simulink model "gcu"  (R2025b)
settings: Solver=FixedStepAuto  StartTime=0.0  StopTime=10.0  RelTol=1e-3
undefined symbols (not defined in the file): controller, luen, quadcop, traj, Ts_gcs, xi0
settings Model: DataDictionary=project.sldd  Creator=Nick  LastModifiedBy=Rakete

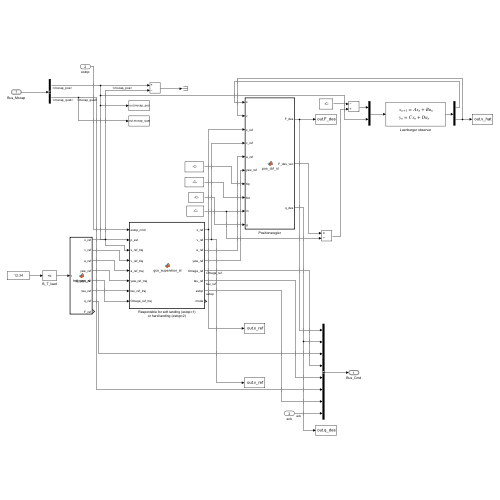
[thumbnail: Simulink's stored preview of the top-level diagram]
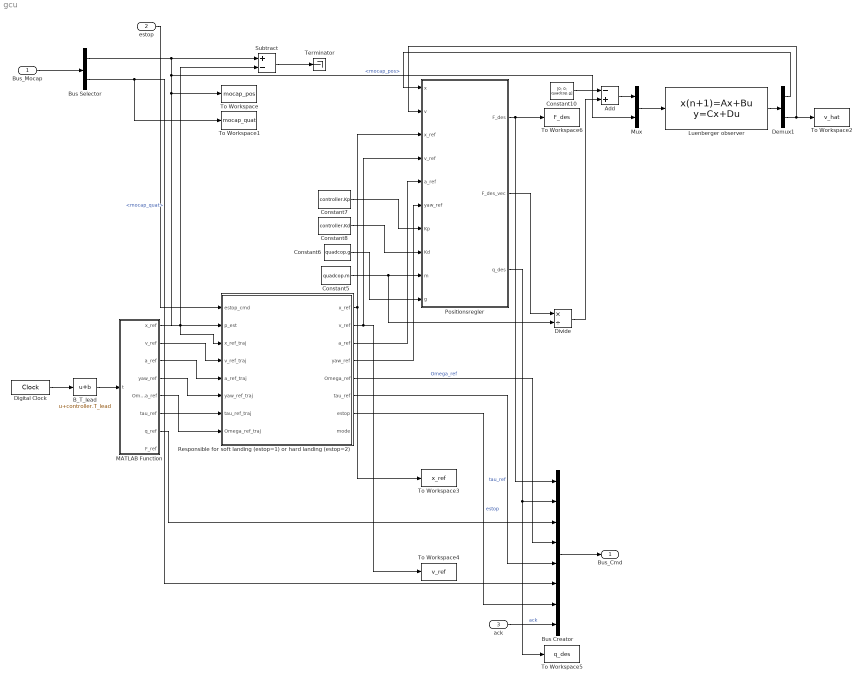
== system gcu ==
  Bus_Mocap : Inport  OutDataTypeStr=Bus: Bus_Mocap
  estop : Inport  Port=2  OutDataTypeStr=uint8
  ack : Inport  Port=3  OutDataTypeStr=boolean  PortDimensions=1
  Add : Sum  Inputs=-+
  B_T_lead : Bias  Bias=controller.T_lead  SaturateOnIntegerOverflow=off
  Bus Creator : BusCreator  Inputs=8  OutDataTypeStr=Bus: Bus_Cmd
      settings: InheritFromInputs=off
  Bus Selector : BusSelector  OutputSignals=mocap_pos,mocap_quat
  Constant10 : Constant  Value=[0; 0; quadcop.g]
  Constant5 : Constant  Value=quadcop.m
  Constant6 : Constant  Value=quadcop.g
  Constant7 : Constant  Value=controller.Kp
  Constant8 : Constant  Value=controller.Kd
  Demux1 : Demux  Outputs=2
  Digital Clock : DigitalClock  SampleTime=Ts_gcs
  Divide : Product  Inputs=*/
  Luenberger observer : DiscreteStateSpace  A=luen.Ad  B=luen.Bd  C=luen.Cd  D=luen.Dd  InitialCondition=xi0  SampleTime=Ts_gcs
  MATLAB Function : MATLAB Function  TreatAsAtomicUnit=on
  Mux : Mux  Inputs=2
  Positionsregler : MATLAB Function  TreatAsAtomicUnit=on
  Responsible for soft landing (estop=1) or hard landing (estop=2) : MATLAB Function  TreatAsAtomicUnit=on  SystemSampleTime=Ts_gcs
  Subtract : Sum  Inputs=+-
  Terminator : Terminator
  To Workspace : ToWorkspace  VariableName=mocap_pos  SaveFormat=Timeseries  SampleTime=Ts_gcs
  To Workspace1 : ToWorkspace  VariableName=mocap_quat  SaveFormat=Timeseries  SampleTime=Ts_gcs
  To Workspace2 : ToWorkspace  VariableName=v_hat  SaveFormat=Timeseries  SampleTime=Ts_gcs
  To Workspace3 : ToWorkspace  VariableName=x_ref  SaveFormat=Timeseries  SampleTime=Ts_gcs
  To Workspace4 : ToWorkspace  VariableName=v_ref  SaveFormat=Timeseries  SampleTime=Ts_gcs
  To Workspace5 : ToWorkspace  VariableName=q_des  SaveFormat=Timeseries  SampleTime=Ts_gcs
  To Workspace6 : ToWorkspace  VariableName=F_des  SaveFormat=Timeseries  SampleTime=Ts_gcs
  Bus_Cmd : Outport  OutDataTypeStr=Bus: Bus_Cmd
  wires:
  Responsible for soft landing (estop=1) or hard landing (estop=2)/7(estop) -> Bus Creator/7  "estop"
  MATLAB Function/2(v_ref) -> Responsible for soft landing (estop=1) or hard landing (estop=2)/4(v_ref_traj)
  Responsible for soft landing (estop=1) or hard landing (estop=2)/3(a_ref) -> Positionsregler/5(a_ref)
  MATLAB Function/6(tau_ref) -> Responsible for soft landing (estop=1) or hard landing (estop=2)/7(tau_ref_traj)
  Digital Clock/1 -> B_T_lead/1
  Bus_Mocap/1 -> Bus Selector/1
  MATLAB Function/1(x_ref) -> Subtract/2, Responsible for soft landing (estop=1) or hard landing (estop=2)/3(x_ref_traj)
  B_T_lead/1 -> MATLAB Function/1(t)
  Add/1 -> Mux/1
  Bus Selector/1 -> Responsible for soft landing (estop=1) or hard landing (estop=2)/2(p_est), To Workspace/1, Mux/2, Subtract/1  "<mocap_pos>"
  Responsible for soft landing (estop=1) or hard landing (estop=2)/6(tau_ref) -> Bus Creator/5  "tau_ref"
  estop/1 -> Responsible for soft landing (estop=1) or hard landing (estop=2)/1(estop_cmd)
  Constant7/1 -> Positionsregler/7(Kp)
  Bus Selector/2 -> Bus Creator/6, To Workspace1/1  "<mocap_quat>"
  MATLAB Function/3(a_ref) -> Responsible for soft landing (estop=1) or hard landing (estop=2)/5(a_ref_traj)
  MATLAB Function/4(yaw_ref) -> Responsible for soft landing (estop=1) or hard landing (estop=2)/6(yaw_ref_traj)
  Responsible for soft landing (estop=1) or hard landing (estop=2)/4(yaw_ref) -> Positionsregler/6(yaw_ref)
  MATLAB Function/5(Omega_ref) -> Responsible for soft landing (estop=1) or hard landing (estop=2)/8(Omega_ref_traj)
  MATLAB Function/7(q_ref) -> Bus Creator/3
  Subtract/1 -> Terminator/1
  Constant8/1 -> Positionsregler/8(Kd)
  Constant6/1 -> Positionsregler/10(g)
  Constant5/1 -> Divide/2, Positionsregler/9(m)
  Responsible for soft landing (estop=1) or hard landing (estop=2)/1(x_ref) -> Positionsregler/3(x_ref), To Workspace3/1
  Responsible for soft landing (estop=1) or hard landing (estop=2)/2(v_ref) -> To Workspace4/1, Positionsregler/4(v_ref)
  Responsible for soft landing (estop=1) or hard landing (estop=2)/5(Omega_ref) -> Bus Creator/4  "Omega_ref"
  Positionsregler/1(F_des) -> Bus Creator/1, To Workspace6/1
  Divide/1 -> Add/2
  Positionsregler/2(F_des_vec) -> Divide/1
  Positionsregler/3(q_des) -> To Workspace5/1, Bus Creator/2
  ack/1 -> Bus Creator/8  "ack"
  Constant10/1 -> Add/1
  Bus Creator/1 -> Bus_Cmd/1
  Mux/1 -> Luenberger observer/1
  Luenberger observer/1 -> Demux1/1
  Demux1/1 -> Positionsregler/1(x)
  Demux1/2 -> Positionsregler/2(v), To Workspace2/1

== matlab function gcu/Positionsregler ==
  data: F_des output; x input; F_des_vec output; v input; x_ref input; v_ref input; a_ref input; yaw_ref input; Kp input; Kd input; m input; g input; q_des output
function [F_des, F_des_vec, q_des] = pos_ctrl_sl(x, v, x_ref, v_ref, a_ref, yaw_ref, Kp, Kd, m, g)
%#codegen
% WRAPPER — code liegt in
% scripts\functions\pos_ctrl.m - dieser Block ruft sie nur auf
[F_des, F_des_vec, q_des] = pos_ctrl(x, v, x_ref, v_ref, a_ref, yaw_ref, Kp, Kd, m, g);
end

== matlab function gcu/MATLAB Function ==
  data: t input; x_ref output; v_ref output; a_ref output; yaw_ref output; Omega_ref output; tau_ref output; q_ref output; F_ref output; traj parameter; quadcop parameter
function [x_ref, v_ref, a_ref, yaw_ref, Omega_ref, tau_ref, q_ref, F_ref] = traj_gen_sl(t, traj, quadcop)
%#codegen
% WRAPPER — code liegt in
% scripts\functions\traj_gen.m - dieser Block ruft sie nur auf
[x_ref, v_ref, a_ref, yaw_ref, Omega_ref, tau_ref, q_ref, F_ref] = traj_gen(t, traj, quadcop);
end

== matlab function gcu/Responsible for soft landing (estop=1) or hard landing (estop=2) ==
  data: estop_cmd input; x_ref output; p_est input; x_ref_traj input; v_ref_traj input; a_ref_traj input; yaw_ref_traj input; v_ref output; a_ref output; yaw_ref output; Omega_ref output; tau_ref output; estop output; mode output; tau_ref_traj input; supervisor parameter; Omega_ref_traj input
function [x_ref, v_ref, a_ref, yaw_ref, Omega_ref, tau_ref, estop, mode] = gcs_supervisor_sl(estop_cmd, p_est, x_ref_traj, v_ref_traj, a_ref_traj, yaw_ref_traj, tau_ref_traj, supervisor, Omega_ref_traj)
%#codegen
% WRAPPER — code liegt in
% scripts\functions\gcs_supervisor.m - dieser Block ruft sie nur auf
[x_ref, v_ref, a_ref, yaw_ref, Omega_ref, tau_ref, estop, mode] = gcs_supervisor(estop_cmd, p_est, x_ref_traj, v_ref_traj, a_ref_traj, yaw_ref_traj, tau_ref_traj, supervisor, Omega_ref_traj);
end
